simulink model "CPU"  (R2021a)
settings: Solver=VariableStepAuto  StartTime=0.0  StopTime=10  RelTol=1e-3
libraries: dspsigops x7
settings Model: Creator=kbhar  LastModifiedBy=kbhar

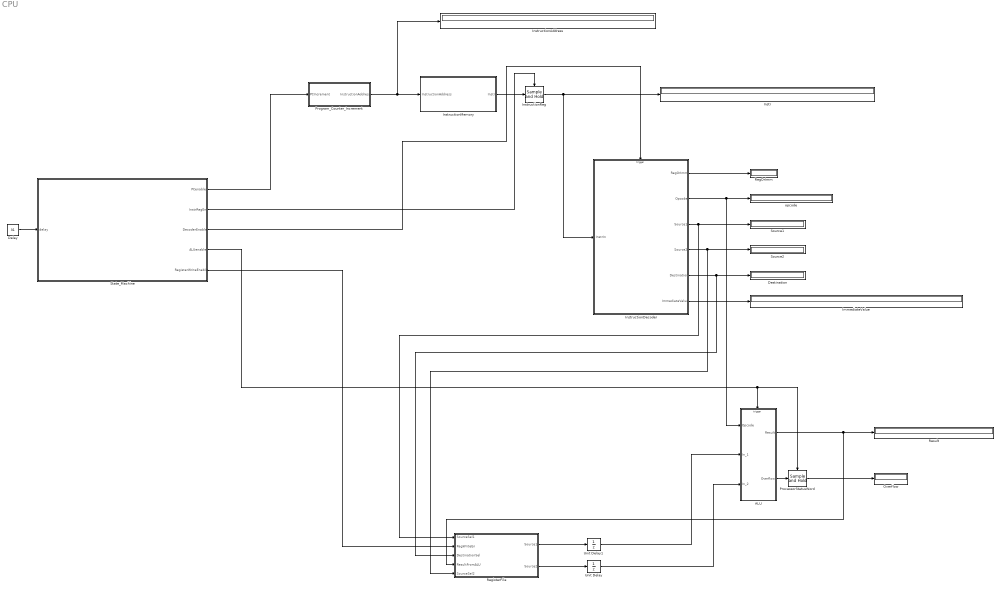
== system CPU ==
  ALU : Subsystem
  Delay : Constant  Value=31
  Destination : Display
  ImmediateValue : Display
  Instr : Display
  InstructionAddress : Display
  InstructionDecoder : Subsystem
  InstructionMemory : Subsystem
  InstructionReg : dspsigops/Sample and Hold  trig=Rising edge  initCond=0  latchinput=off
  Overflow : Display
  ProcessorStatusWord : dspsigops/Sample and Hold  trig=Rising edge  initCond=0  latchinput=off
  Program_Counter_Increment : Subsystem
  RegOrImm : Display
  RegisterFile : Subsystem
  Result : Display
  Source1 : Display
  Source2 : Display
  State_Machine : Stateflow chart  TreatAsAtomicUnit=on
  Unit Delay : UnitDelay  SampleTime=-1  HasFrameUpgradeWarning=on
  Unit Delay1 : UnitDelay  SampleTime=-1  HasFrameUpgradeWarning=on
  opcode : Display
  wires:
  Delay/1 -> State_Machine/1(delay)
  State_Machine/2(InstrRegEn) -> InstructionReg/Trigger
  State_Machine/4(ALUenable) -> ProcessorStatusWord/Trigger, ALU/Trigger
  Unit Delay1/1 -> ALU/2(In_1)
  Unit Delay/1 -> ALU/3(In_2)
  ALU/1(Result) -> RegisterFile/4(ResultFromALU), Result/1
  InstructionDecoder/1(RegOrImm) -> RegOrImm/1
  InstructionDecoder/2(Opcode) -> opcode/1, ALU/1(Opcode)
  InstructionReg/1 -> InstructionDecoder/1(InstrIn), Instr/1
  InstructionDecoder/6(ImmediateValue) -> ImmediateValue/1
  State_Machine/3(DecoderEnable) -> InstructionDecoder/Trigger
  InstructionMemory/1(Instr) -> InstructionReg/1
  Program_Counter_Increment/1(InstructionAddress) -> InstructionAddress/1, InstructionMemory/1(InstructionAddress)
  ALU/2(Overflow) -> ProcessorStatusWord/1
  ProcessorStatusWord/1 -> Overflow/1
  State_Machine/1(PCenable) -> Program_Counter_Increment/1(PCIncrement)
  RegisterFile/1(Source1) -> Unit Delay1/1
  InstructionDecoder/4(Source2) -> RegisterFile/5(SourceSel2), Source2/1
  InstructionDecoder/5(Destination) -> RegisterFile/3(DestinationSel), Destination/1
  State_Machine/5(RegisterWriteEnable) -> RegisterFile/2(RegWriteEn)
  RegisterFile/2(Source2) -> Unit Delay/1
  InstructionDecoder/3(Source1) -> RegisterFile/1(SourceSel1), Source1/1

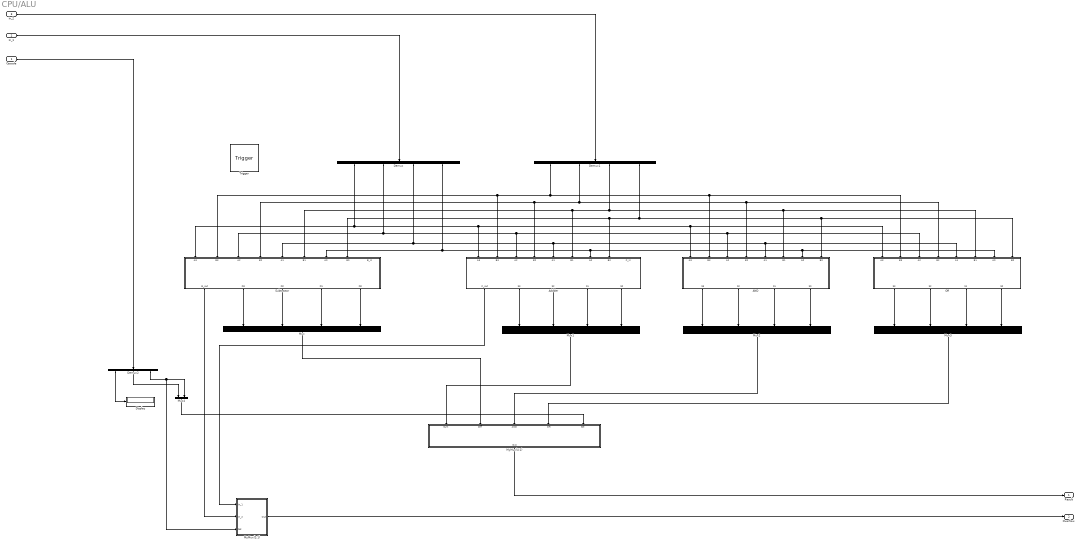
== system CPU/ALU ==
  Opcode : Inport
  In_1 : Inport  Port=2
  In_2 : Inport  Port=3
  Trigger : TriggerPort  VariantControl=(inherit)  PortDimensions=1
  AND : Subsystem
  Addder : Subsystem
  Demux : Demux
  Demux1 : Demux
  Demux2 : Demux  Outputs=3
  Display : Display
  Mux{,1..3} (4 alike) : Mux
  Mux4 : Mux  Inputs=2
  MyMux(2:1) : Subsystem
  MyMux(4:1) : Subsystem
  OR : Subsystem
  Subtractor : Subsystem
  Result : Outport
  Overflow : Outport  Port=2
  wires:
  AND/2(S2) -> Mux2/2
  Demux1/3 -> OR/6(B1), AND/6(B1), Subtractor/6(B1), Addder/6(B1)
  OR/1(S3) -> Mux3/1
  Subtractor/5(D0) -> Mux/4
  OR/3(S1) -> Mux3/3
  Demux1/2 -> OR/4(B2), AND/4(B2), Subtractor/4(B2), Addder/4(B2)
  Mux/1 -> MyMux(4:1)/2(Diff)
  Demux/4 -> Subtractor/7(A0), OR/7(A0), AND/7(A0), Addder/7(A0)
  Addder/3(S2) -> Mux1/2
  Subtractor/2(D3) -> Mux/1
  Demux1/4 -> Subtractor/8(B0), Addder/8(B0), OR/8(B0), AND/8(B0)
  Demux/2 -> Subtractor/3(A2), OR/3(A2), AND/3(A2), Addder/3(A2)
  Demux/1 -> Subtractor/1(A3), OR/1(A3), AND/1(A3), Addder/1(A3)
  MyMux(2:1)/1(Out) -> Overflow/1
  Subtractor/1(B_out) -> MyMux(2:1)/2(In_2)
  Demux1/1 -> OR/2(B3), AND/2(B3), Subtractor/2(B3), Addder/2(B3)
  Demux/3 -> Subtractor/5(A1), AND/5(A1), OR/5(A1), Addder/5(A1)
  MyMux(4:1)/1(Out) -> Result/1
  Subtractor/3(D2) -> Mux/2
  Mux3/1 -> MyMux(4:1)/4(OR)
  Subtractor/4(D1) -> Mux/3
  Mux1/1 -> MyMux(4:1)/1(Sum)
  ? -> Addder/9(C_in)
  AND/1(S3) -> Mux2/1
  Mux2/1 -> MyMux(4:1)/3(AND)
  In_2/1 -> Demux1/1
  OR/2(S2) -> Mux3/2
  Mux4/1 -> MyMux(4:1)/5(Sel)
  AND/4(S0) -> Mux2/4
  Demux2/1 -> Display/1
  Demux2/3 -> MyMux(2:1)/3(Sel), Mux4/2
  Demux2/2 -> Mux4/1
  Addder/1(C_out) -> MyMux(2:1)/1(In_1)
  Addder/4(S1) -> Mux1/3
  AND/3(S1) -> Mux2/3
  Addder/5(S0) -> Mux1/4
  OR/4(S0) -> Mux3/4
  ? -> Subtractor/9(B_in)
  Addder/2(S3) -> Mux1/1
  Opcode/1 -> Demux2/1
  In_1/1 -> Demux/1

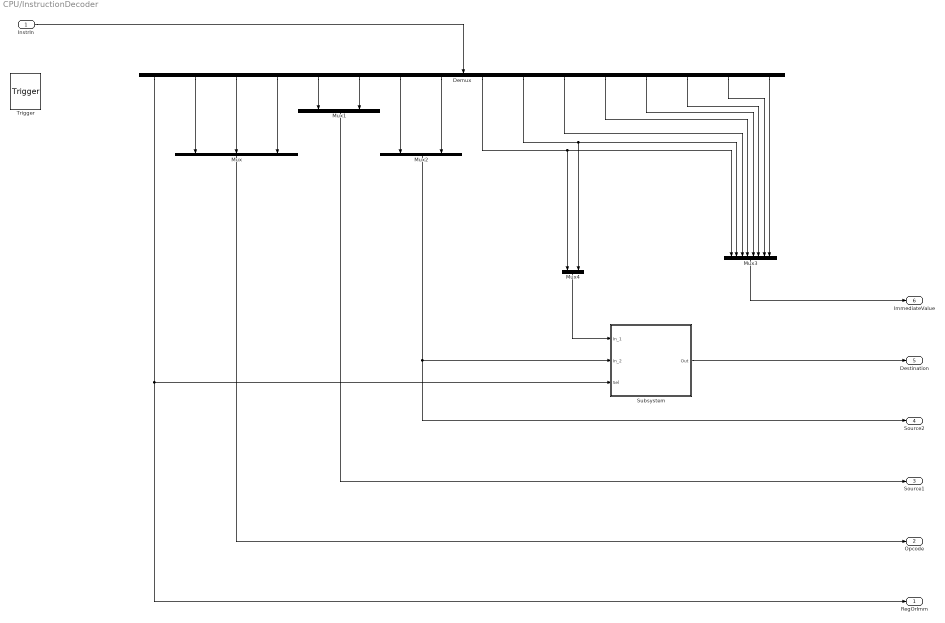
== system CPU/InstructionDecoder ==
  InstrIn : Inport
  Trigger : TriggerPort  VariantControl=(inherit)  PortDimensions=1
  Demux : Demux  Outputs=16
  Mux : Mux  Inputs=3
  Mux1 : Mux  Inputs=2
  Mux2 : Mux  Inputs=2
  Mux3 : Mux  Inputs=8
  Mux4 : Mux  Inputs=2
  Subsystem : Subsystem
  RegOrImm : Outport
  Opcode : Outport  Port=2
  Source1 : Outport  Port=3
  Source2 : Outport  Port=4
  Destination : Outport  Port=5
  ImmediateValue : Outport  Port=6
  wires:
  Demux/4 -> Mux/3
  Mux4/1 -> Subsystem/1(In_1)
  Demux/12 -> Mux3/4
  Demux/9 -> Mux4/1, Mux3/1
  Demux/15 -> Mux3/7
  Demux/13 -> Mux3/5
  Demux/2 -> Mux/1
  Demux/14 -> Mux3/6
  Mux2/1 -> Source2/1, Subsystem/2(In_2)
  Demux/1 -> RegOrImm/1, Subsystem/3(Sel)
  Demux/6 -> Mux1/2
  Demux/5 -> Mux1/1
  Demux/7 -> Mux2/1
  Demux/8 -> Mux2/2
  Demux/10 -> Mux3/2, Mux4/2
  Demux/3 -> Mux/2
  Demux/16 -> Mux3/8
  Demux/11 -> Mux3/3
  Subsystem/1(Out) -> Destination/1
  Mux1/1 -> Source1/1
  InstrIn/1 -> Demux/1
  Mux3/1 -> ImmediateValue/1
  Mux/1 -> Opcode/1

== system CPU/InstructionMemory ==
  InstructionAddress : Inport
  Demux : Demux
  Display{,1..3} (4 alike) : Display
  ImmediateTypeInstruction1 : Constant  Value=[1 0 0 0 0 1 0 0 1 0 0 0 0 0 0 0]
  ImmediateTypeInstruction2 : Constant  Value=[1 0 0 1 0 0 1 1 1 1 0 0 0 0 0 0]
  Mux : Mux  Inputs=2
  MyMux(4:1) : Subsystem
  RegisterTypeInstruction1 : Constant  Value=[0 0 0 0 0 1 1 0 0 1 0 0 0 0 0 0]
  RegisterTypeInstruction2 : Constant  Value=[0 0 0 1 0 0 1 0 1 1 0 0 0 0 0 0]
  Instr : Outport
  wires:
  Mux/1 -> Display2/1, MyMux(4:1)/5(Sel)
  ImmediateTypeInstruction2/1 -> MyMux(4:1)/2(In_2)
  InstructionAddress/1 -> Display3/1, Demux/1
  Demux/4 -> Mux/2
  RegisterTypeInstruction1/1 -> MyMux(4:1)/3(In_3)
  Demux/1 -> Display/1
  Demux/3 -> Mux/1
  Demux/2 -> Display1/1
  ImmediateTypeInstruction1/1 -> MyMux(4:1)/1(In_1)
  RegisterTypeInstruction2/1 -> MyMux(4:1)/4(In_4)
  MyMux(4:1)/1(Out) -> Instr/1

== system CPU/Program_Counter_Increment ==
  PCIncrement : Inport
  Addder : Subsystem
  Constant1 : Constant
  Constant2 : Constant  Value=0
  Demux : Demux
  Display : Display
  Mux : Mux
  ProgramCounter : dspsigops/Sample and Hold  trig=Rising edge  initCond=[0 0 0 0]  latchinput=off
  Unit Delay : UnitDelay  SampleTime=-1  HasFrameUpgradeWarning=on
  InstructionAddress : Outport
  wires:
  Constant2/1 -> Addder/2(B3), Addder/4(B2), Addder/6(B1), Addder/9(C_in)
  Demux/3 -> Addder/5(A1)
  Mux/1 -> InstructionAddress/1, Unit Delay/1
  Addder/4(S1) -> Mux/3
  ProgramCounter/1 -> Demux/1
  Addder/1(C_out) -> Display/1
  Unit Delay/1 -> ProgramCounter/1
  Addder/5(S0) -> Mux/4
  Addder/3(S2) -> Mux/2
  Constant1/1 -> Addder/8(B0)
  Addder/2(S3) -> Mux/1
  Demux/2 -> Addder/3(A2)
  Demux/4 -> Addder/7(A0)
  Demux/1 -> Addder/1(A3)
  PCIncrement/1 -> ProgramCounter/Trigger

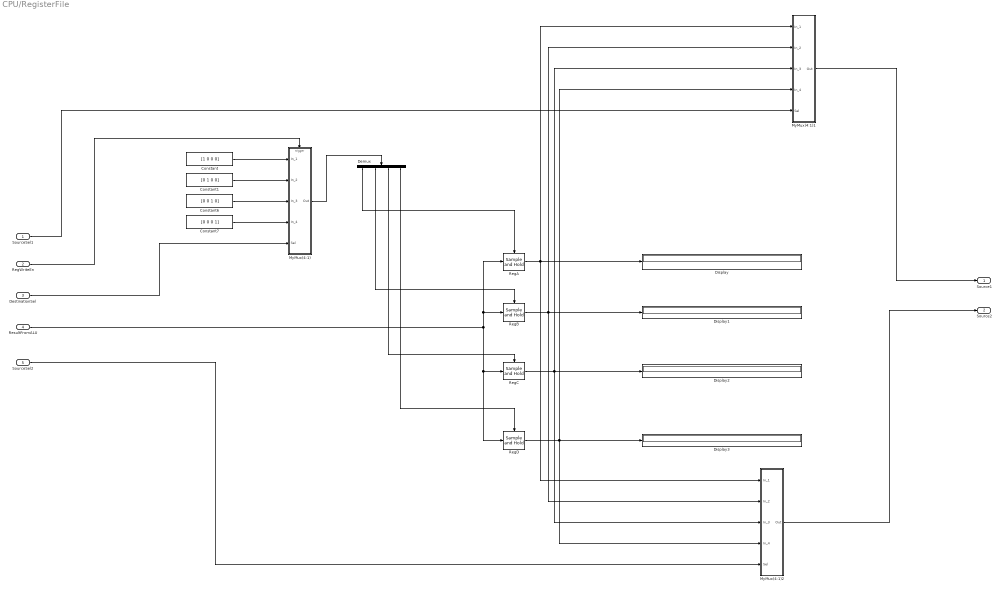
== system CPU/RegisterFile ==
  SourceSel1 : Inport
  RegWriteEn : Inport  Port=2
  DestinationSel : Inport  Port=3
  ResultFromALU : Inport  Port=4
  SourceSel2 : Inport  Port=5
  Constant : Constant  Value=[1 0 0 0]
  Constant1 : Constant  Value=[0 1 0 0]
  Constant6 : Constant  Value=[0 0 1 0]
  Constant7 : Constant  Value=[0 0 0 1]
  Demux : Demux
  Display{,1..3} (4 alike) : Display
  MyMux(4:1) : Subsystem
  MyMux(4:1)1 : Subsystem
  MyMux(4:1)2 : Subsystem
  RegA : dspsigops/Sample and Hold  trig=Rising edge  initCond=[1 1 1 1]  latchinput=off
  RegB : dspsigops/Sample and Hold  trig=Rising edge  initCond=[0 1 0 0]  latchinput=off
  RegC : dspsigops/Sample and Hold  trig=Rising edge  initCond=[0 1 0 1]  latchinput=off
  RegD : dspsigops/Sample and Hold  trig=Rising edge  initCond=[0 0 0 0]  latchinput=off
  Source1 : Outport
  Source2 : Outport  Port=2
  wires:
  ResultFromALU/1 -> RegD/1, RegC/1, RegA/1, RegB/1
  RegB/1 -> MyMux(4:1)2/2(In_2), MyMux(4:1)1/2(In_2), Display1/1
  RegC/1 -> MyMux(4:1)2/3(In_3), MyMux(4:1)1/3(In_3), Display2/1
  Demux/1 -> RegA/Trigger
  RegA/1 -> MyMux(4:1)2/1(In_1), MyMux(4:1)1/1(In_1), Display/1
  Constant7/1 -> MyMux(4:1)/4(In_4)
  RegD/1 -> MyMux(4:1)2/4(In_4), MyMux(4:1)1/4(In_4), Display3/1
  Constant/1 -> MyMux(4:1)/1(In_1)
  Constant6/1 -> MyMux(4:1)/3(In_3)
  Constant1/1 -> MyMux(4:1)/2(In_2)
  Demux/4 -> RegD/Trigger
  SourceSel1/1 -> MyMux(4:1)1/5(Sel)
  Demux/3 -> RegC/Trigger
  MyMux(4:1)1/1(Out) -> Source1/1
  Demux/2 -> RegB/Trigger
  DestinationSel/1 -> MyMux(4:1)/5(Sel)
  MyMux(4:1)/1(Out) -> Demux/1
  RegWriteEn/1 -> MyMux(4:1)/Trigger
  SourceSel2/1 -> MyMux(4:1)2/5(Sel)
  MyMux(4:1)2/1(Out) -> Source2/1

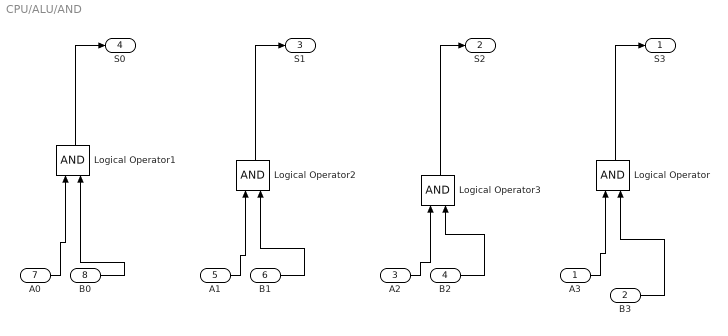
== system CPU/ALU/AND ==
  A3 : Inport
  B3 : Inport  Port=2
  A2 : Inport  Port=3
  B2 : Inport  Port=4
  A1 : Inport  Port=5
  B1 : Inport  Port=6
  A0 : Inport  Port=7
  B0 : Inport  Port=8
  Logical Operator{,1..3} (4 alike) : Logic  AllPortsSameDT=off  OutDataTypeStr=boolean
  S3 : Outport
  S2 : Outport  Port=2
  S1 : Outport  Port=3
  S0 : Outport  Port=4
  wires:
  Logical Operator2/1 -> S1/1
  B1/1 -> Logical Operator2/2
  A1/1 -> Logical Operator2/1
  A2/1 -> Logical Operator3/1
  B0/1 -> Logical Operator1/2
  B3/1 -> Logical Operator/2
  B2/1 -> Logical Operator3/2
  A0/1 -> Logical Operator1/1
  A3/1 -> Logical Operator/1
  Logical Operator3/1 -> S2/1
  Logical Operator1/1 -> S0/1
  Logical Operator/1 -> S3/1

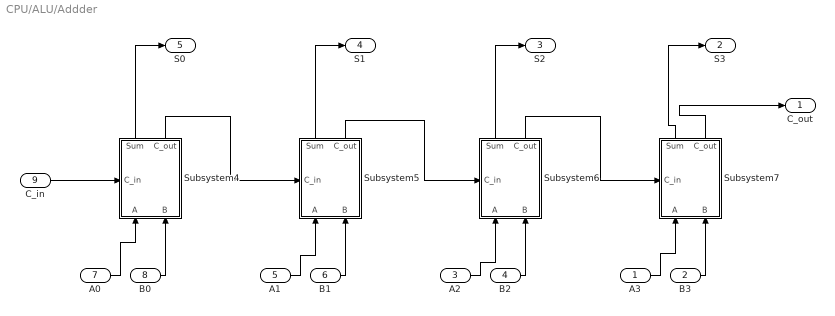
== system CPU/ALU/Addder ==
  A3 : Inport
  B3 : Inport  Port=2
  A2 : Inport  Port=3
  B2 : Inport  Port=4
  A1 : Inport  Port=5
  B1 : Inport  Port=6
  A0 : Inport  Port=7
  B0 : Inport  Port=8
  C_in : Inport  Port=9
  Subsystem4 : Subsystem
      settings: PortSchema="{\"entries\":[{\"content\":{\"sides\":[{\"content\":{\"connectorIds\":[\"In1\",\"In2\"]},\"type\":\"ConnectorPlacement.EquallySpacedRectSide\",\"uuid\":\"38d1d783-1e84-469f-b88f-34400794f458\"},{\"content\":{\"connectorIds\":[\"Out1\",\"Out2\"],\"side\":\"RIGHT\"},\"type\":\"ConnectorPlacement.EquallySpacedRectSide\",\"uuid\":\"9549b396-3b16-432f-9c12-dae7a5b8dc11\"},{\"content\":{\"connectorIds\":[\"In3\"],\"side\":\"TOP\"},\"type\":\"ConnectorPlacement.EquallySpacedRectSide\",\"uuid\":\"526a5790-86b3-4626-b4aa-b9520108ec40\"}]},\"type\":\"ConnectorPlacement.EquallySpacedConnector\",\"uuid\":\"b57ea0ad-738f-4734-9daa-a65058de1f48\"}],\"packageUris\":[\"http://schema.mathworks.com/mf0/Connector/R2020b\"],\"version\":\"1.0\"}"
  Subsystem5 : Subsystem
      settings: PortSchema="{\"entries\":[{\"content\":{\"sides\":[{\"content\":{\"connectorIds\":[\"In1\",\"In2\"]},\"type\":\"ConnectorPlacement.EquallySpacedRectSide\",\"uuid\":\"38d1d783-1e84-469f-b88f-34400794f458\"},{\"content\":{\"connectorIds\":[\"Out1\",\"Out2\"],\"side\":\"RIGHT\"},\"type\":\"ConnectorPlacement.EquallySpacedRectSide\",\"uuid\":\"9549b396-3b16-432f-9c12-dae7a5b8dc11\"},{\"content\":{\"connectorIds\":[\"In3\"],\"side\":\"TOP\"},\"type\":\"ConnectorPlacement.EquallySpacedRectSide\",\"uuid\":\"526a5790-86b3-4626-b4aa-b9520108ec40\"}]},\"type\":\"ConnectorPlacement.EquallySpacedConnector\",\"uuid\":\"b57ea0ad-738f-4734-9daa-a65058de1f48\"}],\"packageUris\":[\"http://schema.mathworks.com/mf0/Connector/R2020b\"],\"version\":\"1.0\"}"
  Subsystem6 : Subsystem
      settings: PortSchema="{\"entries\":[{\"content\":{\"sides\":[{\"content\":{\"connectorIds\":[\"In1\",\"In2\"]},\"type\":\"ConnectorPlacement.EquallySpacedRectSide\",\"uuid\":\"38d1d783-1e84-469f-b88f-34400794f458\"},{\"content\":{\"connectorIds\":[\"Out1\",\"Out2\"],\"side\":\"RIGHT\"},\"type\":\"ConnectorPlacement.EquallySpacedRectSide\",\"uuid\":\"9549b396-3b16-432f-9c12-dae7a5b8dc11\"},{\"content\":{\"connectorIds\":[\"In3\"],\"side\":\"TOP\"},\"type\":\"ConnectorPlacement.EquallySpacedRectSide\",\"uuid\":\"526a5790-86b3-4626-b4aa-b9520108ec40\"}]},\"type\":\"ConnectorPlacement.EquallySpacedConnector\",\"uuid\":\"b57ea0ad-738f-4734-9daa-a65058de1f48\"}],\"packageUris\":[\"http://schema.mathworks.com/mf0/Connector/R2020b\"],\"version\":\"1.0\"}"
  Subsystem7 : Subsystem
      settings: PortSchema="{\"entries\":[{\"content\":{\"sides\":[{\"content\":{\"connectorIds\":[\"In1\",\"In2\"]},\"type\":\"ConnectorPlacement.EquallySpacedRectSide\",\"uuid\":\"38d1d783-1e84-469f-b88f-34400794f458\"},{\"content\":{\"connectorIds\":[\"Out1\",\"Out2\"],\"side\":\"RIGHT\"},\"type\":\"ConnectorPlacement.EquallySpacedRectSide\",\"uuid\":\"9549b396-3b16-432f-9c12-dae7a5b8dc11\"},{\"content\":{\"connectorIds\":[\"In3\"],\"side\":\"TOP\"},\"type\":\"ConnectorPlacement.EquallySpacedRectSide\",\"uuid\":\"526a5790-86b3-4626-b4aa-b9520108ec40\"}]},\"type\":\"ConnectorPlacement.EquallySpacedConnector\",\"uuid\":\"b57ea0ad-738f-4734-9daa-a65058de1f48\"}],\"packageUris\":[\"http://schema.mathworks.com/mf0/Connector/R2020b\"],\"version\":\"1.0\"}"
  C_out : Outport
  S3 : Outport  Port=2
  S2 : Outport  Port=3
  S1 : Outport  Port=4
  S0 : Outport  Port=5
  wires:
  Subsystem5/2(C_out) -> Subsystem6/3(C_in)
  Subsystem5/1(Sum) -> S1/1
  Subsystem7/2(C_out) -> C_out/1
  B1/1 -> Subsystem5/2(B)
  Subsystem6/2(C_out) -> Subsystem7/3(C_in)
  A1/1 -> Subsystem5/1(A)
  A2/1 -> Subsystem6/1(A)
  Subsystem4/2(C_out) -> Subsystem5/3(C_in)
  B0/1 -> Subsystem4/2(B)
  B3/1 -> Subsystem7/2(B)
  B2/1 -> Subsystem6/2(B)
  A0/1 -> Subsystem4/1(A)
  A3/1 -> Subsystem7/1(A)
  Subsystem6/1(Sum) -> S2/1
  C_in/1 -> Subsystem4/3(C_in)
  Subsystem4/1(Sum) -> S0/1
  Subsystem7/1(Sum) -> S3/1

== system CPU/ALU/MyMux(2:1) ==
  In_1 : Inport
  In_2 : Inport  Port=2
  Sel : Inport  Port=3
  Logical Operator : Logic  AllPortsSameDT=off  OutDataTypeStr=boolean
  Logical Operator1 : Logic  Operator=NOT  AllPortsSameDT=off  OutDataTypeStr=boolean
  Logical Operator2 : Logic  AllPortsSameDT=off  OutDataTypeStr=boolean
  Logical Operator3 : Logic  Operator=OR  AllPortsSameDT=off  OutDataTypeStr=boolean
  Out : Outport
  wires:
  Logical Operator1/1 -> Logical Operator/2
  In_1/1 -> Logical Operator/1
  Logical Operator2/1 -> Logical Operator3/2
  Sel/1 -> Logical Operator1/1, Logical Operator2/2
  Logical Operator3/1 -> Out/1
  In_2/1 -> Logical Operator2/1
  Logical Operator/1 -> Logical Operator3/1

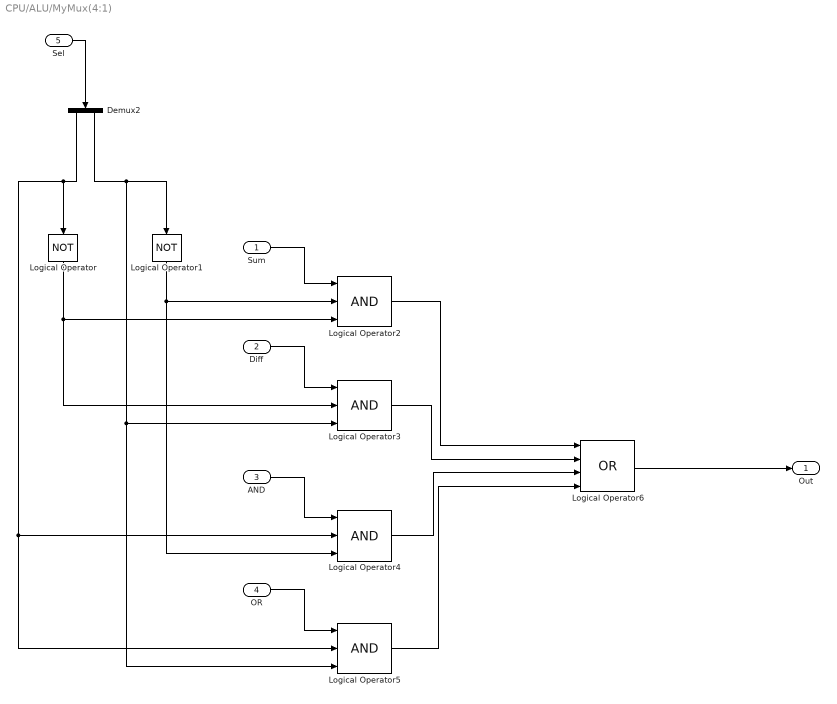
== system CPU/ALU/MyMux(4:1) ==
  Sum : Inport
  Diff : Inport  Port=2
  AND : Inport  Port=3
  OR : Inport  Port=4
  Sel : Inport  Port=5
  Demux2 : Demux  Outputs=2
  Logical Operator : Logic  Operator=NOT  AllPortsSameDT=off  OutDataTypeStr=boolean
  Logical Operator1 : Logic  Operator=NOT  AllPortsSameDT=off  OutDataTypeStr=boolean
  Logical Operator{2..5} (4 alike) : Logic  Inputs=3  AllPortsSameDT=off  OutDataTypeStr=boolean
  Logical Operator6 : Logic  Operator=OR  Inputs=4  AllPortsSameDT=off  OutDataTypeStr=boolean
  Out : Outport
  wires:
  Demux2/1 -> Logical Operator4/2, Logical Operator5/2, Logical Operator/1
  Demux2/2 -> Logical Operator5/3, Logical Operator3/3, Logical Operator1/1
  Logical Operator1/1 -> Logical Operator2/2, Logical Operator4/3
  Logical Operator2/1 -> Logical Operator6/1
  Logical Operator3/1 -> Logical Operator6/2
  Logical Operator/1 -> Logical Operator2/3, Logical Operator3/2
  Logical Operator4/1 -> Logical Operator6/3
  Logical Operator5/1 -> Logical Operator6/4
  Diff/1 -> Logical Operator3/1
  AND/1 -> Logical Operator4/1
  OR/1 -> Logical Operator5/1
  Sum/1 -> Logical Operator2/1
  Logical Operator6/1 -> Out/1
  Sel/1 -> Demux2/1

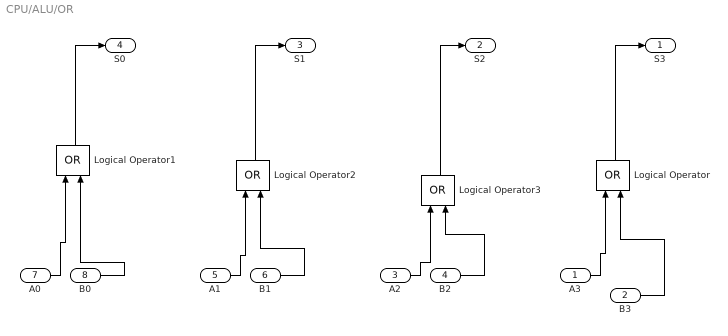
== system CPU/ALU/OR ==
  A3 : Inport
  B3 : Inport  Port=2
  A2 : Inport  Port=3
  B2 : Inport  Port=4
  A1 : Inport  Port=5
  B1 : Inport  Port=6
  A0 : Inport  Port=7
  B0 : Inport  Port=8
  Logical Operator{,1..3} (4 alike) : Logic  Operator=OR  AllPortsSameDT=off  OutDataTypeStr=boolean
  S3 : Outport
  S2 : Outport  Port=2
  S1 : Outport  Port=3
  S0 : Outport  Port=4
  wires:
  Logical Operator2/1 -> S1/1
  B1/1 -> Logical Operator2/2
  A1/1 -> Logical Operator2/1
  A2/1 -> Logical Operator3/1
  B0/1 -> Logical Operator1/2
  B3/1 -> Logical Operator/2
  B2/1 -> Logical Operator3/2
  A0/1 -> Logical Operator1/1
  A3/1 -> Logical Operator/1
  Logical Operator3/1 -> S2/1
  Logical Operator1/1 -> S0/1
  Logical Operator/1 -> S3/1

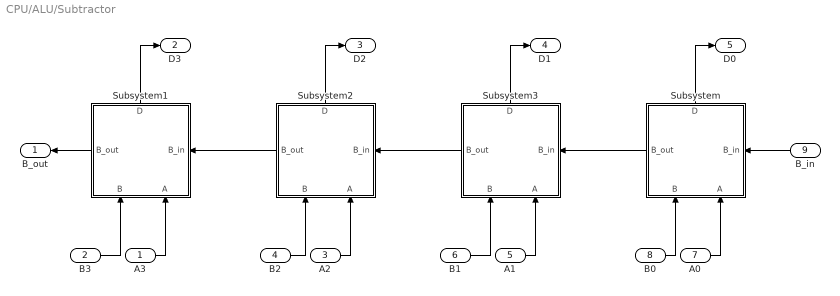
== system CPU/ALU/Subtractor ==
  A3 : Inport
  B3 : Inport  Port=2
  A2 : Inport  Port=3
  B2 : Inport  Port=4
  A1 : Inport  Port=5
  B1 : Inport  Port=6
  A0 : Inport  Port=7
  B0 : Inport  Port=8
  B_in : Inport  Port=9
  Subsystem : Subsystem
      settings: PortSchema="{\"entries\":[{\"content\":{\"sides\":[{\"content\":{\"connectorIds\":[\"In1\",\"In2\"]},\"type\":\"ConnectorPlacement.EquallySpacedRectSide\",\"uuid\":\"38d1d783-1e84-469f-b88f-34400794f458\"},{\"content\":{\"connectorIds\":[\"Out1\"],\"side\":\"RIGHT\"},\"type\":\"ConnectorPlacement.EquallySpacedRectSide\",\"uuid\":\"9549b396-3b16-432f-9c12-dae7a5b8dc11\"},{\"content\":{\"connectorIds\":[\"Out2\"],\"side\":\"TOP\"},\"type\":\"ConnectorPlacement.EquallySpacedRectSide\",\"uuid\":\"526a5790-86b3-4626-b4aa-b9520108ec40\"},{\"content\":{\"connectorIds\":[\"In3\"],\"side\":\"BOTTOM\"},\"type\":\"ConnectorPlacement.EquallySpacedRectSide\",\"uuid\":\"7b9a1b6a-14be-425f-b6da-6563ee756159\"}]},\"type\":\"ConnectorPlacement.EquallySpacedConnector\",\"uuid\":\"b57ea0ad-738f-4734-9daa-a65058de1f48\"}],\"packageUris\":[\"http://schema.mathworks.com/mf0/Connector/R2020b\"],\"version\":\"1.0\"}"
  Subsystem1 : Subsystem
      settings: PortSchema="{\"entries\":[{\"content\":{\"sides\":[{\"content\":{\"connectorIds\":[\"In1\",\"In2\"]},\"type\":\"ConnectorPlacement.EquallySpacedRectSide\",\"uuid\":\"38d1d783-1e84-469f-b88f-34400794f458\"},{\"content\":{\"connectorIds\":[\"Out1\"],\"side\":\"RIGHT\"},\"type\":\"ConnectorPlacement.EquallySpacedRectSide\",\"uuid\":\"9549b396-3b16-432f-9c12-dae7a5b8dc11\"},{\"content\":{\"connectorIds\":[\"Out2\"],\"side\":\"TOP\"},\"type\":\"ConnectorPlacement.EquallySpacedRectSide\",\"uuid\":\"526a5790-86b3-4626-b4aa-b9520108ec40\"},{\"content\":{\"connectorIds\":[\"In3\"],\"side\":\"BOTTOM\"},\"type\":\"ConnectorPlacement.EquallySpacedRectSide\",\"uuid\":\"7b9a1b6a-14be-425f-b6da-6563ee756159\"}]},\"type\":\"ConnectorPlacement.EquallySpacedConnector\",\"uuid\":\"b57ea0ad-738f-4734-9daa-a65058de1f48\"}],\"packageUris\":[\"http://schema.mathworks.com/mf0/Connector/R2020b\"],\"version\":\"1.0\"}"
  Subsystem2 : Subsystem
      settings: PortSchema="{\"entries\":[{\"content\":{\"sides\":[{\"content\":{\"connectorIds\":[\"In1\",\"In2\"]},\"type\":\"ConnectorPlacement.EquallySpacedRectSide\",\"uuid\":\"38d1d783-1e84-469f-b88f-34400794f458\"},{\"content\":{\"connectorIds\":[\"Out1\"],\"side\":\"RIGHT\"},\"type\":\"ConnectorPlacement.EquallySpacedRectSide\",\"uuid\":\"9549b396-3b16-432f-9c12-dae7a5b8dc11\"},{\"content\":{\"connectorIds\":[\"Out2\"],\"side\":\"TOP\"},\"type\":\"ConnectorPlacement.EquallySpacedRectSide\",\"uuid\":\"526a5790-86b3-4626-b4aa-b9520108ec40\"},{\"content\":{\"connectorIds\":[\"In3\"],\"side\":\"BOTTOM\"},\"type\":\"ConnectorPlacement.EquallySpacedRectSide\",\"uuid\":\"7b9a1b6a-14be-425f-b6da-6563ee756159\"}]},\"type\":\"ConnectorPlacement.EquallySpacedConnector\",\"uuid\":\"b57ea0ad-738f-4734-9daa-a65058de1f48\"}],\"packageUris\":[\"http://schema.mathworks.com/mf0/Connector/R2020b\"],\"version\":\"1.0\"}"
  Subsystem3 : Subsystem
      settings: PortSchema="{\"entries\":[{\"content\":{\"sides\":[{\"content\":{\"connectorIds\":[\"In1\",\"In2\"]},\"type\":\"ConnectorPlacement.EquallySpacedRectSide\",\"uuid\":\"38d1d783-1e84-469f-b88f-34400794f458\"},{\"content\":{\"connectorIds\":[\"Out1\"],\"side\":\"RIGHT\"},\"type\":\"ConnectorPlacement.EquallySpacedRectSide\",\"uuid\":\"9549b396-3b16-432f-9c12-dae7a5b8dc11\"},{\"content\":{\"connectorIds\":[\"Out2\"],\"side\":\"TOP\"},\"type\":\"ConnectorPlacement.EquallySpacedRectSide\",\"uuid\":\"526a5790-86b3-4626-b4aa-b9520108ec40\"},{\"content\":{\"connectorIds\":[\"In3\"],\"side\":\"BOTTOM\"},\"type\":\"ConnectorPlacement.EquallySpacedRectSide\",\"uuid\":\"7b9a1b6a-14be-425f-b6da-6563ee756159\"}]},\"type\":\"ConnectorPlacement.EquallySpacedConnector\",\"uuid\":\"b57ea0ad-738f-4734-9daa-a65058de1f48\"}],\"packageUris\":[\"http://schema.mathworks.com/mf0/Connector/R2020b\"],\"version\":\"1.0\"}"
  B_out : Outport
  D3 : Outport  Port=2
  D2 : Outport  Port=3
  D1 : Outport  Port=4
  D0 : Outport  Port=5
  wires:
  B_in/1 -> Subsystem/3(B_in)
  Subsystem3/2(B_out) -> Subsystem2/3(B_in)
  Subsystem2/2(B_out) -> Subsystem1/3(B_in)
  Subsystem/2(B_out) -> Subsystem3/3(B_in)
  Subsystem1/2(B_out) -> B_out/1
  A0/1 -> Subsystem/2(A)
  B0/1 -> Subsystem/1(B)
  B3/1 -> Subsystem1/1(B)
  A3/1 -> Subsystem1/2(A)
  A1/1 -> Subsystem3/2(A)
  B1/1 -> Subsystem3/1(B)
  B2/1 -> Subsystem2/1(B)
  A2/1 -> Subsystem2/2(A)
  Subsystem1/1(D) -> D3/1
  Subsystem/1(D) -> D0/1
  Subsystem3/1(D) -> D1/1
  Subsystem2/1(D) -> D2/1

== system CPU/InstructionDecoder/Subsystem ==
  In_1 : Inport
  In_2 : Inport  Port=2
  Sel : Inport  Port=3
  Logical Operator : Logic  AllPortsSameDT=off  OutDataTypeStr=boolean
  Logical Operator1 : Logic  Operator=NOT  AllPortsSameDT=off  OutDataTypeStr=boolean
  Logical Operator2 : Logic  AllPortsSameDT=off  OutDataTypeStr=boolean
  Logical Operator3 : Logic  Operator=OR  AllPortsSameDT=off  OutDataTypeStr=boolean
  Out : Outport
  wires:
  Logical Operator/1 -> Logical Operator3/1
  Logical Operator1/1 -> Logical Operator/2
  Sel/1 -> Logical Operator1/1, Logical Operator2/2
  Logical Operator2/1 -> Logical Operator3/2
  In_2/1 -> Logical Operator2/1
  In_1/1 -> Logical Operator/1
  Logical Operator3/1 -> Out/1

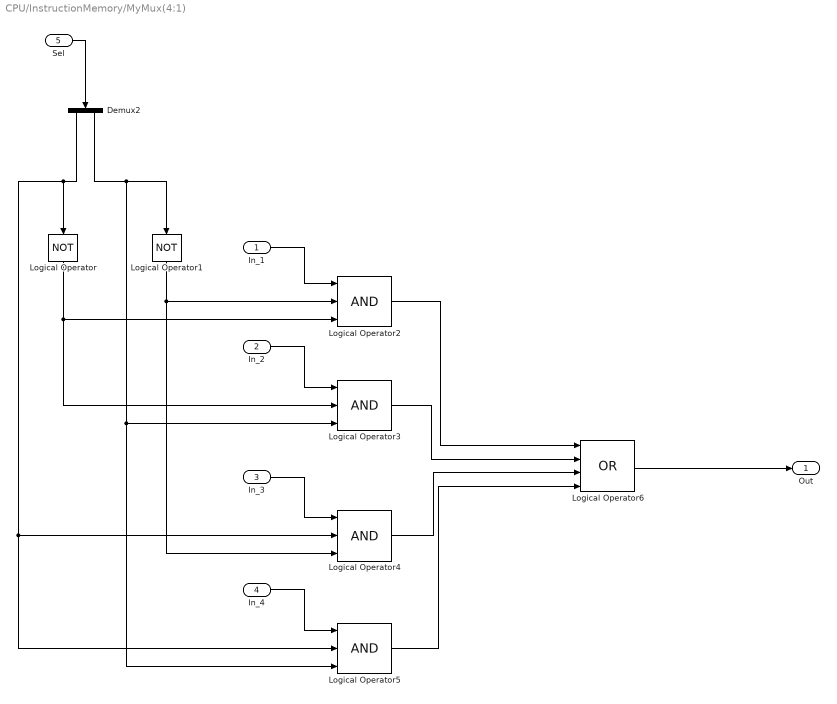
== system CPU/InstructionMemory/MyMux(4:1) ==
  In_1 : Inport
  In_2 : Inport  Port=2
  In_3 : Inport  Port=3
  In_4 : Inport  Port=4
  Sel : Inport  Port=5
  Demux2 : Demux  Outputs=2
  Logical Operator : Logic  Operator=NOT  AllPortsSameDT=off  OutDataTypeStr=boolean
  Logical Operator1 : Logic  Operator=NOT  AllPortsSameDT=off  OutDataTypeStr=boolean
  Logical Operator{2..5} (4 alike) : Logic  Inputs=3  AllPortsSameDT=off  OutDataTypeStr=boolean
  Logical Operator6 : Logic  Operator=OR  Inputs=4  AllPortsSameDT=off  OutDataTypeStr=boolean
  Out : Outport
  wires:
  Demux2/1 -> Logical Operator4/2, Logical Operator5/2, Logical Operator/1
  Demux2/2 -> Logical Operator5/3, Logical Operator3/3, Logical Operator1/1
  Logical Operator1/1 -> Logical Operator2/2, Logical Operator4/3
  Logical Operator2/1 -> Logical Operator6/1
  Logical Operator3/1 -> Logical Operator6/2
  Logical Operator/1 -> Logical Operator2/3, Logical Operator3/2
  Logical Operator4/1 -> Logical Operator6/3
  Logical Operator5/1 -> Logical Operator6/4
  In_2/1 -> Logical Operator3/1
  In_3/1 -> Logical Operator4/1
  In_4/1 -> Logical Operator5/1
  In_1/1 -> Logical Operator2/1
  Logical Operator6/1 -> Out/1
  Sel/1 -> Demux2/1

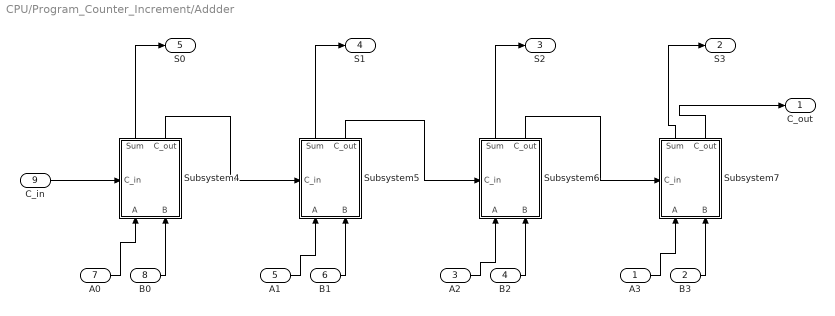
== system CPU/Program_Counter_Increment/Addder ==
  A3 : Inport
  B3 : Inport  Port=2
  A2 : Inport  Port=3
  B2 : Inport  Port=4
  A1 : Inport  Port=5
  B1 : Inport  Port=6
  A0 : Inport  Port=7
  B0 : Inport  Port=8
  C_in : Inport  Port=9
  Subsystem4 : Subsystem
      settings: PortSchema="{\"entries\":[{\"content\":{\"sides\":[{\"content\":{\"connectorIds\":[\"In1\",\"In2\"]},\"type\":\"ConnectorPlacement.EquallySpacedRectSide\",\"uuid\":\"38d1d783-1e84-469f-b88f-34400794f458\"},{\"content\":{\"connectorIds\":[\"Out1\",\"Out2\"],\"side\":\"RIGHT\"},\"type\":\"ConnectorPlacement.EquallySpacedRectSide\",\"uuid\":\"9549b396-3b16-432f-9c12-dae7a5b8dc11\"},{\"content\":{\"connectorIds\":[\"In3\"],\"side\":\"TOP\"},\"type\":\"ConnectorPlacement.EquallySpacedRectSide\",\"uuid\":\"526a5790-86b3-4626-b4aa-b9520108ec40\"}]},\"type\":\"ConnectorPlacement.EquallySpacedConnector\",\"uuid\":\"b57ea0ad-738f-4734-9daa-a65058de1f48\"}],\"packageUris\":[\"http://schema.mathworks.com/mf0/Connector/R2020b\"],\"version\":\"1.0\"}"
  Subsystem5 : Subsystem
      settings: PortSchema="{\"entries\":[{\"content\":{\"sides\":[{\"content\":{\"connectorIds\":[\"In1\",\"In2\"]},\"type\":\"ConnectorPlacement.EquallySpacedRectSide\",\"uuid\":\"38d1d783-1e84-469f-b88f-34400794f458\"},{\"content\":{\"connectorIds\":[\"Out1\",\"Out2\"],\"side\":\"RIGHT\"},\"type\":\"ConnectorPlacement.EquallySpacedRectSide\",\"uuid\":\"9549b396-3b16-432f-9c12-dae7a5b8dc11\"},{\"content\":{\"connectorIds\":[\"In3\"],\"side\":\"TOP\"},\"type\":\"ConnectorPlacement.EquallySpacedRectSide\",\"uuid\":\"526a5790-86b3-4626-b4aa-b9520108ec40\"}]},\"type\":\"ConnectorPlacement.EquallySpacedConnector\",\"uuid\":\"b57ea0ad-738f-4734-9daa-a65058de1f48\"}],\"packageUris\":[\"http://schema.mathworks.com/mf0/Connector/R2020b\"],\"version\":\"1.0\"}"
  Subsystem6 : Subsystem
      settings: PortSchema="{\"entries\":[{\"content\":{\"sides\":[{\"content\":{\"connectorIds\":[\"In1\",\"In2\"]},\"type\":\"ConnectorPlacement.EquallySpacedRectSide\",\"uuid\":\"38d1d783-1e84-469f-b88f-34400794f458\"},{\"content\":{\"connectorIds\":[\"Out1\",\"Out2\"],\"side\":\"RIGHT\"},\"type\":\"ConnectorPlacement.EquallySpacedRectSide\",\"uuid\":\"9549b396-3b16-432f-9c12-dae7a5b8dc11\"},{\"content\":{\"connectorIds\":[\"In3\"],\"side\":\"TOP\"},\"type\":\"ConnectorPlacement.EquallySpacedRectSide\",\"uuid\":\"526a5790-86b3-4626-b4aa-b9520108ec40\"}]},\"type\":\"ConnectorPlacement.EquallySpacedConnector\",\"uuid\":\"b57ea0ad-738f-4734-9daa-a65058de1f48\"}],\"packageUris\":[\"http://schema.mathworks.com/mf0/Connector/R2020b\"],\"version\":\"1.0\"}"
  Subsystem7 : Subsystem
      settings: PortSchema="{\"entries\":[{\"content\":{\"sides\":[{\"content\":{\"connectorIds\":[\"In1\",\"In2\"]},\"type\":\"ConnectorPlacement.EquallySpacedRectSide\",\"uuid\":\"38d1d783-1e84-469f-b88f-34400794f458\"},{\"content\":{\"connectorIds\":[\"Out1\",\"Out2\"],\"side\":\"RIGHT\"},\"type\":\"ConnectorPlacement.EquallySpacedRectSide\",\"uuid\":\"9549b396-3b16-432f-9c12-dae7a5b8dc11\"},{\"content\":{\"connectorIds\":[\"In3\"],\"side\":\"TOP\"},\"type\":\"ConnectorPlacement.EquallySpacedRectSide\",\"uuid\":\"526a5790-86b3-4626-b4aa-b9520108ec40\"}]},\"type\":\"ConnectorPlacement.EquallySpacedConnector\",\"uuid\":\"b57ea0ad-738f-4734-9daa-a65058de1f48\"}],\"packageUris\":[\"http://schema.mathworks.com/mf0/Connector/R2020b\"],\"version\":\"1.0\"}"
  C_out : Outport
  S3 : Outport  Port=2
  S2 : Outport  Port=3
  S1 : Outport  Port=4
  S0 : Outport  Port=5
  wires:
  Subsystem5/2(C_out) -> Subsystem6/3(C_in)
  Subsystem5/1(Sum) -> S1/1
  Subsystem7/2(C_out) -> C_out/1
  B1/1 -> Subsystem5/2(B)
  Subsystem6/2(C_out) -> Subsystem7/3(C_in)
  A1/1 -> Subsystem5/1(A)
  A2/1 -> Subsystem6/1(A)
  Subsystem4/2(C_out) -> Subsystem5/3(C_in)
  B0/1 -> Subsystem4/2(B)
  B3/1 -> Subsystem7/2(B)
  B2/1 -> Subsystem6/2(B)
  A0/1 -> Subsystem4/1(A)
  A3/1 -> Subsystem7/1(A)
  Subsystem6/1(Sum) -> S2/1
  C_in/1 -> Subsystem4/3(C_in)
  Subsystem4/1(Sum) -> S0/1
  Subsystem7/1(Sum) -> S3/1

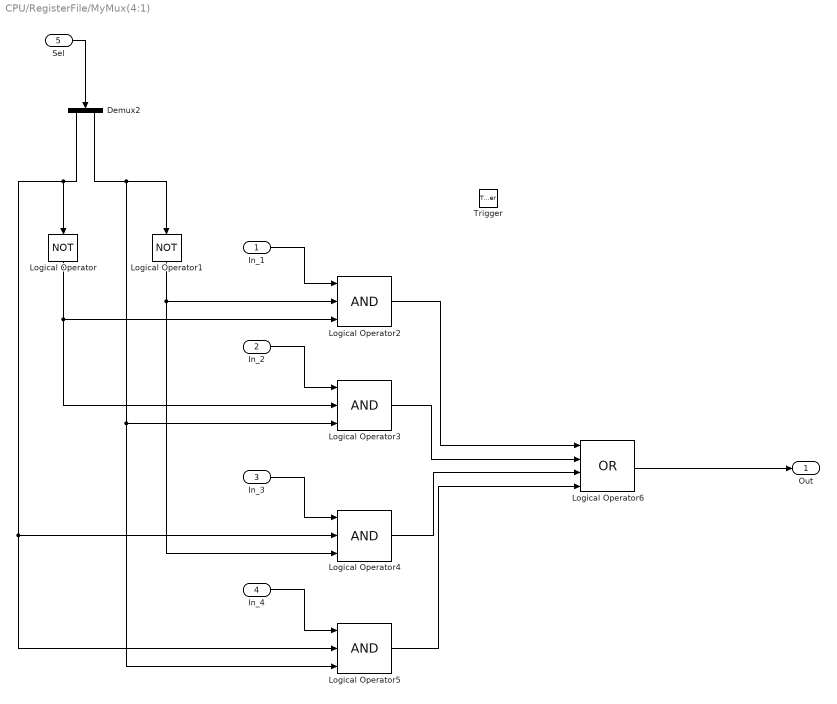
== system CPU/RegisterFile/MyMux(4:1) ==
  In_1 : Inport
  In_2 : Inport  Port=2
  In_3 : Inport  Port=3
  In_4 : Inport  Port=4
  Sel : Inport  Port=5
  Trigger : TriggerPort  VariantControl=(inherit)  PortDimensions=1
  Demux2 : Demux  Outputs=2
  Logical Operator : Logic  Operator=NOT  AllPortsSameDT=off  OutDataTypeStr=boolean
  Logical Operator1 : Logic  Operator=NOT  AllPortsSameDT=off  OutDataTypeStr=boolean
  Logical Operator{2..5} (4 alike) : Logic  Inputs=3  AllPortsSameDT=off  OutDataTypeStr=boolean
  Logical Operator6 : Logic  Operator=OR  Inputs=4  AllPortsSameDT=off  OutDataTypeStr=boolean
  Out : Outport
  wires:
  Demux2/1 -> Logical Operator4/2, Logical Operator5/2, Logical Operator/1
  Demux2/2 -> Logical Operator5/3, Logical Operator3/3, Logical Operator1/1
  Logical Operator1/1 -> Logical Operator2/2, Logical Operator4/3
  Logical Operator2/1 -> Logical Operator6/1
  Logical Operator3/1 -> Logical Operator6/2
  Logical Operator/1 -> Logical Operator2/3, Logical Operator3/2
  Logical Operator4/1 -> Logical Operator6/3
  Logical Operator5/1 -> Logical Operator6/4
  In_2/1 -> Logical Operator3/1
  In_3/1 -> Logical Operator4/1
  In_4/1 -> Logical Operator5/1
  In_1/1 -> Logical Operator2/1
  Logical Operator6/1 -> Out/1
  Sel/1 -> Demux2/1

== system CPU/RegisterFile/MyMux(4:1)1 ==
  In_1 : Inport
  In_2 : Inport  Port=2
  In_3 : Inport  Port=3
  In_4 : Inport  Port=4
  Sel : Inport  Port=5
  Demux2 : Demux  Outputs=2
  Logical Operator : Logic  Operator=NOT  AllPortsSameDT=off  OutDataTypeStr=boolean
  Logical Operator1 : Logic  Operator=NOT  AllPortsSameDT=off  OutDataTypeStr=boolean
  Logical Operator{2..5} (4 alike) : Logic  Inputs=3  AllPortsSameDT=off  OutDataTypeStr=boolean
  Logical Operator6 : Logic  Operator=OR  Inputs=4  AllPortsSameDT=off  OutDataTypeStr=boolean
  Out : Outport
  wires:
  Demux2/1 -> Logical Operator4/2, Logical Operator5/2, Logical Operator/1
  Demux2/2 -> Logical Operator5/3, Logical Operator3/3, Logical Operator1/1
  Logical Operator1/1 -> Logical Operator2/2, Logical Operator4/3
  Logical Operator2/1 -> Logical Operator6/1
  Logical Operator3/1 -> Logical Operator6/2
  Logical Operator/1 -> Logical Operator2/3, Logical Operator3/2
  Logical Operator4/1 -> Logical Operator6/3
  Logical Operator5/1 -> Logical Operator6/4
  In_2/1 -> Logical Operator3/1
  In_3/1 -> Logical Operator4/1
  In_4/1 -> Logical Operator5/1
  In_1/1 -> Logical Operator2/1
  Logical Operator6/1 -> Out/1
  Sel/1 -> Demux2/1

== system CPU/RegisterFile/MyMux(4:1)2 ==
  In_1 : Inport
  In_2 : Inport  Port=2
  In_3 : Inport  Port=3
  In_4 : Inport  Port=4
  Sel : Inport  Port=5
  Demux2 : Demux  Outputs=2
  Logical Operator : Logic  Operator=NOT  AllPortsSameDT=off  OutDataTypeStr=boolean
  Logical Operator1 : Logic  Operator=NOT  AllPortsSameDT=off  OutDataTypeStr=boolean
  Logical Operator{2..5} (4 alike) : Logic  Inputs=3  AllPortsSameDT=off  OutDataTypeStr=boolean
  Logical Operator6 : Logic  Operator=OR  Inputs=4  AllPortsSameDT=off  OutDataTypeStr=boolean
  Out : Outport
  wires:
  Demux2/1 -> Logical Operator4/2, Logical Operator5/2, Logical Operator/1
  Demux2/2 -> Logical Operator5/3, Logical Operator3/3, Logical Operator1/1
  Logical Operator1/1 -> Logical Operator2/2, Logical Operator4/3
  Logical Operator2/1 -> Logical Operator6/1
  Logical Operator3/1 -> Logical Operator6/2
  Logical Operator/1 -> Logical Operator2/3, Logical Operator3/2
  Logical Operator4/1 -> Logical Operator6/3
  Logical Operator5/1 -> Logical Operator6/4
  In_2/1 -> Logical Operator3/1
  In_3/1 -> Logical Operator4/1
  In_4/1 -> Logical Operator5/1
  In_1/1 -> Logical Operator2/1
  Logical Operator6/1 -> Out/1
  Sel/1 -> Demux2/1

== system CPU/ALU/Addder/Subsystem4 ==
  A : Inport
  B : Inport  Port=2
  C_in : Inport  Port=3
  Logical Operator : Logic  Operator=XOR  AllPortsSameDT=off  OutDataTypeStr=boolean
  Logical Operator1 : Logic  Operator=OR  AllPortsSameDT=off  OutDataTypeStr=boolean
  Logical Operator2 : Logic  Operator=XOR  AllPortsSameDT=off  OutDataTypeStr=boolean
  Logical Operator3 : Logic  AllPortsSameDT=off  OutDataTypeStr=boolean
  Logical Operator4 : Logic  AllPortsSameDT=off  OutDataTypeStr=boolean
  Sum : Outport
  C_out : Outport  Port=2
  wires:
  B/1 -> Logical Operator3/2, Logical Operator2/2
  A/1 -> Logical Operator3/1, Logical Operator2/1
  Logical Operator4/1 -> Logical Operator1/1
  Logical Operator/1 -> Sum/1
  Logical Operator2/1 -> Logical Operator4/1, Logical Operator/1
  C_in/1 -> Logical Operator4/2, Logical Operator/2
  Logical Operator3/1 -> Logical Operator1/2
  Logical Operator1/1 -> C_out/1

== system CPU/ALU/Addder/Subsystem5 ==
  A : Inport
  B : Inport  Port=2
  C_in : Inport  Port=3
  Logical Operator : Logic  Operator=XOR  AllPortsSameDT=off  OutDataTypeStr=boolean
  Logical Operator1 : Logic  Operator=OR  AllPortsSameDT=off  OutDataTypeStr=boolean
  Logical Operator2 : Logic  Operator=XOR  AllPortsSameDT=off  OutDataTypeStr=boolean
  Logical Operator3 : Logic  AllPortsSameDT=off  OutDataTypeStr=boolean
  Logical Operator4 : Logic  AllPortsSameDT=off  OutDataTypeStr=boolean
  Sum : Outport
  C_out : Outport  Port=2
  wires:
  B/1 -> Logical Operator3/2, Logical Operator2/2
  A/1 -> Logical Operator3/1, Logical Operator2/1
  Logical Operator4/1 -> Logical Operator1/1
  Logical Operator/1 -> Sum/1
  Logical Operator2/1 -> Logical Operator4/1, Logical Operator/1
  C_in/1 -> Logical Operator4/2, Logical Operator/2
  Logical Operator3/1 -> Logical Operator1/2
  Logical Operator1/1 -> C_out/1

== system CPU/ALU/Addder/Subsystem6 ==
  A : Inport
  B : Inport  Port=2
  C_in : Inport  Port=3
  Logical Operator : Logic  Operator=XOR  AllPortsSameDT=off  OutDataTypeStr=boolean
  Logical Operator1 : Logic  Operator=OR  AllPortsSameDT=off  OutDataTypeStr=boolean
  Logical Operator2 : Logic  Operator=XOR  AllPortsSameDT=off  OutDataTypeStr=boolean
  Logical Operator3 : Logic  AllPortsSameDT=off  OutDataTypeStr=boolean
  Logical Operator4 : Logic  AllPortsSameDT=off  OutDataTypeStr=boolean
  Sum : Outport
  C_out : Outport  Port=2
  wires:
  B/1 -> Logical Operator3/2, Logical Operator2/2
  A/1 -> Logical Operator3/1, Logical Operator2/1
  Logical Operator4/1 -> Logical Operator1/1
  Logical Operator/1 -> Sum/1
  Logical Operator2/1 -> Logical Operator4/1, Logical Operator/1
  C_in/1 -> Logical Operator4/2, Logical Operator/2
  Logical Operator3/1 -> Logical Operator1/2
  Logical Operator1/1 -> C_out/1

== system CPU/ALU/Addder/Subsystem7 ==
  A : Inport
  B : Inport  Port=2
  C_in : Inport  Port=3
  Logical Operator : Logic  Operator=XOR  AllPortsSameDT=off  OutDataTypeStr=boolean
  Logical Operator1 : Logic  Operator=OR  AllPortsSameDT=off  OutDataTypeStr=boolean
  Logical Operator2 : Logic  Operator=XOR  AllPortsSameDT=off  OutDataTypeStr=boolean
  Logical Operator3 : Logic  AllPortsSameDT=off  OutDataTypeStr=boolean
  Logical Operator4 : Logic  AllPortsSameDT=off  OutDataTypeStr=boolean
  Sum : Outport
  C_out : Outport  Port=2
  wires:
  B/1 -> Logical Operator3/2, Logical Operator2/2
  A/1 -> Logical Operator3/1, Logical Operator2/1
  Logical Operator4/1 -> Logical Operator1/1
  Logical Operator/1 -> Sum/1
  Logical Operator2/1 -> Logical Operator4/1, Logical Operator/1
  C_in/1 -> Logical Operator4/2, Logical Operator/2
  Logical Operator3/1 -> Logical Operator1/2
  Logical Operator1/1 -> C_out/1

== system CPU/ALU/Subtractor/Subsystem ==
  B : Inport
  A : Inport  Port=2
  B_in : Inport  Port=3
  Logical Operator : Logic  Operator=XOR  AllPortsSameDT=off  OutDataTypeStr=boolean
  Logical Operator1 : Logic  Operator=XOR  AllPortsSameDT=off  OutDataTypeStr=boolean
  Logical Operator2 : Logic  Operator=NOT  AllPortsSameDT=off  OutDataTypeStr=boolean
  Logical Operator3 : Logic  AllPortsSameDT=off  OutDataTypeStr=boolean
  Logical Operator4 : Logic  Operator=NOT  AllPortsSameDT=off  OutDataTypeStr=boolean
  Logical Operator5 : Logic  AllPortsSameDT=off  OutDataTypeStr=boolean
  Logical Operator8 : Logic  Operator=OR  AllPortsSameDT=off  OutDataTypeStr=boolean
  D : Outport
  B_out : Outport  Port=2
  wires:
  Logical Operator2/1 -> Logical Operator3/1
  B_in/1 -> Logical Operator/1, Logical Operator3/2
  B/1 -> Logical Operator1/2, Logical Operator5/2
  Logical Operator1/1 -> Logical Operator2/1, Logical Operator/2
  A/1 -> Logical Operator1/1, Logical Operator4/1
  Logical Operator3/1 -> Logical Operator8/1
  Logical Operator5/1 -> Logical Operator8/2
  Logical Operator4/1 -> Logical Operator5/1
  Logical Operator/1 -> D/1
  Logical Operator8/1 -> B_out/1

== system CPU/ALU/Subtractor/Subsystem1 ==
  B : Inport
  A : Inport  Port=2
  B_in : Inport  Port=3
  Logical Operator : Logic  Operator=XOR  AllPortsSameDT=off  OutDataTypeStr=boolean
  Logical Operator1 : Logic  Operator=XOR  AllPortsSameDT=off  OutDataTypeStr=boolean
  Logical Operator2 : Logic  Operator=NOT  AllPortsSameDT=off  OutDataTypeStr=boolean
  Logical Operator3 : Logic  AllPortsSameDT=off  OutDataTypeStr=boolean
  Logical Operator4 : Logic  Operator=NOT  AllPortsSameDT=off  OutDataTypeStr=boolean
  Logical Operator5 : Logic  AllPortsSameDT=off  OutDataTypeStr=boolean
  Logical Operator8 : Logic  Operator=OR  AllPortsSameDT=off  OutDataTypeStr=boolean
  D : Outport
  B_out : Outport  Port=2
  wires:
  Logical Operator2/1 -> Logical Operator3/1
  B_in/1 -> Logical Operator/1, Logical Operator3/2
  B/1 -> Logical Operator1/2, Logical Operator5/2
  Logical Operator1/1 -> Logical Operator2/1, Logical Operator/2
  A/1 -> Logical Operator1/1, Logical Operator4/1
  Logical Operator3/1 -> Logical Operator8/1
  Logical Operator5/1 -> Logical Operator8/2
  Logical Operator4/1 -> Logical Operator5/1
  Logical Operator/1 -> D/1
  Logical Operator8/1 -> B_out/1

== system CPU/ALU/Subtractor/Subsystem2 ==
  B : Inport
  A : Inport  Port=2
  B_in : Inport  Port=3
  Logical Operator : Logic  Operator=XOR  AllPortsSameDT=off  OutDataTypeStr=boolean
  Logical Operator1 : Logic  Operator=XOR  AllPortsSameDT=off  OutDataTypeStr=boolean
  Logical Operator2 : Logic  Operator=NOT  AllPortsSameDT=off  OutDataTypeStr=boolean
  Logical Operator3 : Logic  AllPortsSameDT=off  OutDataTypeStr=boolean
  Logical Operator4 : Logic  Operator=NOT  AllPortsSameDT=off  OutDataTypeStr=boolean
  Logical Operator5 : Logic  AllPortsSameDT=off  OutDataTypeStr=boolean
  Logical Operator8 : Logic  Operator=OR  AllPortsSameDT=off  OutDataTypeStr=boolean
  D : Outport
  B_out : Outport  Port=2
  wires:
  Logical Operator2/1 -> Logical Operator3/1
  B_in/1 -> Logical Operator/1, Logical Operator3/2
  B/1 -> Logical Operator1/2, Logical Operator5/2
  Logical Operator1/1 -> Logical Operator2/1, Logical Operator/2
  A/1 -> Logical Operator1/1, Logical Operator4/1
  Logical Operator3/1 -> Logical Operator8/1
  Logical Operator5/1 -> Logical Operator8/2
  Logical Operator4/1 -> Logical Operator5/1
  Logical Operator/1 -> D/1
  Logical Operator8/1 -> B_out/1

== system CPU/ALU/Subtractor/Subsystem3 ==
  B : Inport
  A : Inport  Port=2
  B_in : Inport  Port=3
  Logical Operator : Logic  Operator=XOR  AllPortsSameDT=off  OutDataTypeStr=boolean
  Logical Operator1 : Logic  Operator=XOR  AllPortsSameDT=off  OutDataTypeStr=boolean
  Logical Operator2 : Logic  Operator=NOT  AllPortsSameDT=off  OutDataTypeStr=boolean
  Logical Operator3 : Logic  AllPortsSameDT=off  OutDataTypeStr=boolean
  Logical Operator4 : Logic  Operator=NOT  AllPortsSameDT=off  OutDataTypeStr=boolean
  Logical Operator5 : Logic  AllPortsSameDT=off  OutDataTypeStr=boolean
  Logical Operator8 : Logic  Operator=OR  AllPortsSameDT=off  OutDataTypeStr=boolean
  D : Outport
  B_out : Outport  Port=2
  wires:
  Logical Operator2/1 -> Logical Operator3/1
  B_in/1 -> Logical Operator/1, Logical Operator3/2
  B/1 -> Logical Operator1/2, Logical Operator5/2
  Logical Operator1/1 -> Logical Operator2/1, Logical Operator/2
  A/1 -> Logical Operator1/1, Logical Operator4/1
  Logical Operator3/1 -> Logical Operator8/1
  Logical Operator5/1 -> Logical Operator8/2
  Logical Operator4/1 -> Logical Operator5/1
  Logical Operator/1 -> D/1
  Logical Operator8/1 -> B_out/1

== system CPU/Program_Counter_Increment/Addder/Subsystem4 ==
  A : Inport
  B : Inport  Port=2
  C_in : Inport  Port=3
  Logical Operator : Logic  Operator=XOR  AllPortsSameDT=off  OutDataTypeStr=boolean
  Logical Operator1 : Logic  Operator=OR  AllPortsSameDT=off  OutDataTypeStr=boolean
  Logical Operator2 : Logic  Operator=XOR  AllPortsSameDT=off  OutDataTypeStr=boolean
  Logical Operator3 : Logic  AllPortsSameDT=off  OutDataTypeStr=boolean
  Logical Operator4 : Logic  AllPortsSameDT=off  OutDataTypeStr=boolean
  Sum : Outport
  C_out : Outport  Port=2
  wires:
  B/1 -> Logical Operator3/2, Logical Operator2/2
  A/1 -> Logical Operator3/1, Logical Operator2/1
  Logical Operator4/1 -> Logical Operator1/1
  Logical Operator/1 -> Sum/1
  Logical Operator2/1 -> Logical Operator4/1, Logical Operator/1
  C_in/1 -> Logical Operator4/2, Logical Operator/2
  Logical Operator3/1 -> Logical Operator1/2
  Logical Operator1/1 -> C_out/1

== system CPU/Program_Counter_Increment/Addder/Subsystem5 ==
  A : Inport
  B : Inport  Port=2
  C_in : Inport  Port=3
  Logical Operator : Logic  Operator=XOR  AllPortsSameDT=off  OutDataTypeStr=boolean
  Logical Operator1 : Logic  Operator=OR  AllPortsSameDT=off  OutDataTypeStr=boolean
  Logical Operator2 : Logic  Operator=XOR  AllPortsSameDT=off  OutDataTypeStr=boolean
  Logical Operator3 : Logic  AllPortsSameDT=off  OutDataTypeStr=boolean
  Logical Operator4 : Logic  AllPortsSameDT=off  OutDataTypeStr=boolean
  Sum : Outport
  C_out : Outport  Port=2
  wires:
  B/1 -> Logical Operator3/2, Logical Operator2/2
  A/1 -> Logical Operator3/1, Logical Operator2/1
  Logical Operator4/1 -> Logical Operator1/1
  Logical Operator/1 -> Sum/1
  Logical Operator2/1 -> Logical Operator4/1, Logical Operator/1
  C_in/1 -> Logical Operator4/2, Logical Operator/2
  Logical Operator3/1 -> Logical Operator1/2
  Logical Operator1/1 -> C_out/1

== system CPU/Program_Counter_Increment/Addder/Subsystem6 ==
  A : Inport
  B : Inport  Port=2
  C_in : Inport  Port=3
  Logical Operator : Logic  Operator=XOR  AllPortsSameDT=off  OutDataTypeStr=boolean
  Logical Operator1 : Logic  Operator=OR  AllPortsSameDT=off  OutDataTypeStr=boolean
  Logical Operator2 : Logic  Operator=XOR  AllPortsSameDT=off  OutDataTypeStr=boolean
  Logical Operator3 : Logic  AllPortsSameDT=off  OutDataTypeStr=boolean
  Logical Operator4 : Logic  AllPortsSameDT=off  OutDataTypeStr=boolean
  Sum : Outport
  C_out : Outport  Port=2
  wires:
  B/1 -> Logical Operator3/2, Logical Operator2/2
  A/1 -> Logical Operator3/1, Logical Operator2/1
  Logical Operator4/1 -> Logical Operator1/1
  Logical Operator/1 -> Sum/1
  Logical Operator2/1 -> Logical Operator4/1, Logical Operator/1
  C_in/1 -> Logical Operator4/2, Logical Operator/2
  Logical Operator3/1 -> Logical Operator1/2
  Logical Operator1/1 -> C_out/1

== system CPU/Program_Counter_Increment/Addder/Subsystem7 ==
  A : Inport
  B : Inport  Port=2
  C_in : Inport  Port=3
  Logical Operator : Logic  Operator=XOR  AllPortsSameDT=off  OutDataTypeStr=boolean
  Logical Operator1 : Logic  Operator=OR  AllPortsSameDT=off  OutDataTypeStr=boolean
  Logical Operator2 : Logic  Operator=XOR  AllPortsSameDT=off  OutDataTypeStr=boolean
  Logical Operator3 : Logic  AllPortsSameDT=off  OutDataTypeStr=boolean
  Logical Operator4 : Logic  AllPortsSameDT=off  OutDataTypeStr=boolean
  Sum : Outport
  C_out : Outport  Port=2
  wires:
  B/1 -> Logical Operator3/2, Logical Operator2/2
  A/1 -> Logical Operator3/1, Logical Operator2/1
  Logical Operator4/1 -> Logical Operator1/1
  Logical Operator/1 -> Sum/1
  Logical Operator2/1 -> Logical Operator4/1, Logical Operator/1
  C_in/1 -> Logical Operator4/2, Logical Operator/2
  Logical Operator3/1 -> Logical Operator1/2
  Logical Operator1/1 -> C_out/1

== stateflow chart CPU/State_Machine ==
  state start
    PCenable = 0; InstrRegEn = 0; DecoderEnable = 0; ALUenable = 0; RegisterWriteEnable = 0;
  state Fetch
    PCenable = 1; InstrRegEn = 1; DecoderEnable = 0; ALUenable = 0; RegisterWriteEnable = 0;
  state Decode
    PCenable = 0; InstrRegEn = 0; DecoderEnable = 1; ALUenable = 0; RegisterWriteEnable = 0;
  state Execute
    PCenable = 0; InstrRegEn = 0; DecoderEnable = 0; ALUenable = 1; RegisterWriteEnable = 0;
  state Writeback
    PCenable = 0; InstrRegEn = 0; DecoderEnable = 0; ALUenable = 0; RegisterWriteEnable = 1;
  (default) -> start
  start -> Fetch
  Writeback -> Fetch : [delay > 40]
  Fetch -> Decode : [delay > 10]
  Decode -> Execute : [delay > 20]
  Execute -> Writeback : [delay > 30]
  data: delay input; PCenable output; InstrRegEn output; DecoderEnable output; ALUenable output; RegisterWriteEnable output
